simulink subsystem "Sensors"  (R2024b)
settings: Solver=VariableStepAuto  StartTime=0.0  StopTime=10.0  RelTol=1e-3
values from neighbouring files (symbols this model uses):
  CurrentFaultSwitch = 0    [Data__MOTOR.m]    (also in Generator_Data.m = 1; Generator_Datatest.m)
  rate_noise_i = 0.02*In    (= 0.22)    [Data__MOTOR.m]    (also in Generator_Data.m = 0.02; Generator_Datatest.m)
  rate_noise_w = 0.02*Wn    (= 2.96)    [Data__MOTOR.m]    (also in Generator_Data.m = 0.002; Generator_Datatest.m)
undefined symbols (not defined in the file or in its folder): sigbuilder_block
settings Model: Creator=Nasser  LastModifiedBy=Nasser

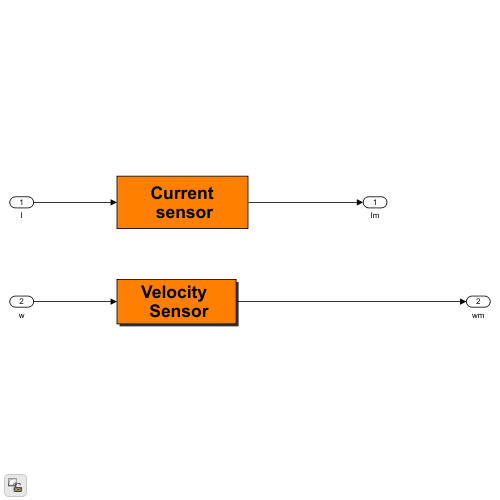
[thumbnail: Simulink's stored preview of the top-level diagram]
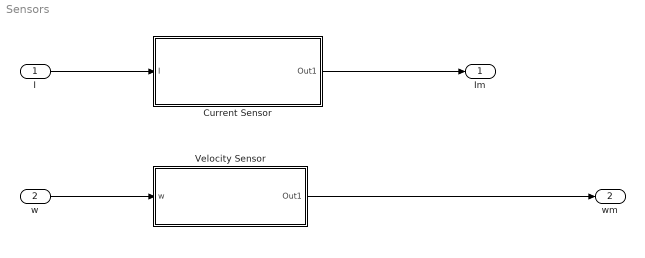
== system Sensors ==
  I : Inport
  w : Inport  Port=2
  Current Sensor : Subsystem
      mask Display: disp('Current\n sensor')
  Velocity Sensor : Subsystem
      mask Display: disp('Velocity \n Sensor')
  Im : Outport
  wm : Outport  Port=2
  wires:
  I/1 -> Current Sensor/1(I)
  w/1 -> Velocity Sensor/1(w)
  Current Sensor/1(Out1) -> Im/1
  Velocity Sensor/1(Out1) -> wm/1

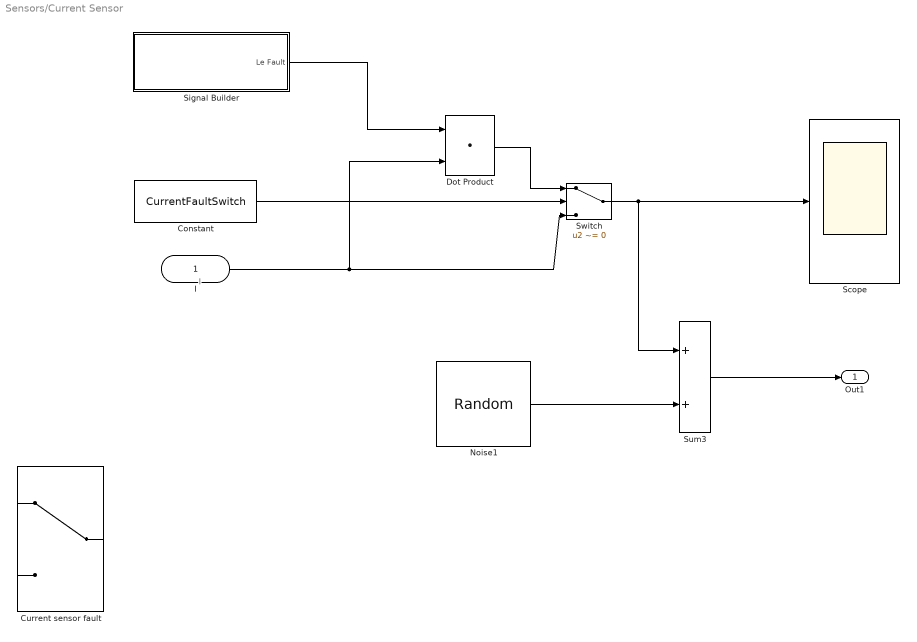
== system Sensors/Current Sensor ==
  note: I
  I : Inport
  Constant : Constant  Value=CurrentFaultSwitch
  Current sensor fault : ManualSwitch
  Dot Product : DotProduct  OutDataTypeStr=Inherit: Inherit via internal rule
  Noise1 : UniformRandomNumber  Minimum=-rate_noise_i  Maximum=+rate_noise_i  SampleTime=0.1
  Scope : Scope
  Signal Builder : Subsystem  Tag=STV Subsys  LoadFcn=sigbuilder_block('load');  StartFcn=sigbuilder_block('start');  StopFcn=sigbuilder_block('stop');  ClipboardFcn=sigbuilder_block('clipboard');  mask(Sigbuilder block){tuvar=[0:10]}
      mask help: Simulink:masks:SigbuilderBlock_MD
      mask init:
      | if ~strcmp(get_param(bdroot(gcbh),'SimulationStatus'),'stopped') tuvar = sigbuilder_block('maskInit'); end
      settings: CopyFcn=sigbuilder_block('copy');  DeleteFcn=sigbuilder_block('delete');  ModelCloseFcn=sigbuilder_block('modelClose');  PreSaveFcn=sigbuilder_block('preSave');  PauseFcn=sigbuilder_block('pause');  ContinueFcn=sigbuilder_block('continue');  NameChangeFcn=sigbuilder_block('namechange');  OpenFcn=sigbuilder_block('open',[1280 104 1024 485.5 ]);  CloseFcn=sigbuilder_block('close');
      mask Display: plot(0, 0, 100, 100,[2, 2, 32, 32, 2], [68, 8, 8, 68, 68],[32, 2], [38, 38], [32, 19, 2],[53, 60, 44], [32, 17, 17, 2],[16, 16, 31, 31]);txt = getActiveGroup(gcbh);text(2, 100, txt,'verticalAlignment', 'top');
  Sum3 : Sum  InputSameDT=on  SaturateOnIntegerOverflow=on  OutDataTypeStr=Inherit: Same as first input
  Switch : Switch  Criteria=u2 ~= 0  Threshold=1  SaturateOnIntegerOverflow=off  InputSameDT=off
  Out1 : Outport  VectorParamsAs1DForOutWhenUnconnected=off
  wires:
  Switch/1 -> Sum3/1, Scope/1
  Constant/1 -> Switch/2
  Dot Product/1 -> Switch/1
  Signal Builder/1(Le Fault) -> Dot Product/1
  I/1 -> Switch/3, Dot Product/2
  Noise1/1 -> Sum3/2
  Sum3/1 -> Out1/1

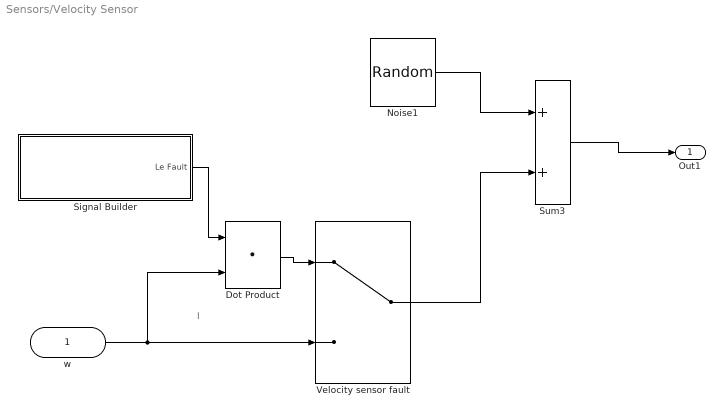
== system Sensors/Velocity Sensor ==
  note: I
  w : Inport
  Dot Product : DotProduct  OutDataTypeStr=Inherit: Inherit via internal rule
  Noise1 : UniformRandomNumber  Minimum=-rate_noise_w  Maximum=+rate_noise_w  SampleTime=0.1
  Signal Builder : Subsystem  Tag=STV Subsys  LoadFcn=sigbuilder_block('load');  StartFcn=sigbuilder_block('start');  StopFcn=sigbuilder_block('stop');  ClipboardFcn=sigbuilder_block('clipboard');  mask(Sigbuilder block){tuvar=[0:10]}
      mask help: Simulink:masks:SigbuilderBlock_MD
      mask init:
      | if ~strcmp(get_param(bdroot(gcbh),'SimulationStatus'),'stopped') tuvar = sigbuilder_block('maskInit'); end
      settings: CopyFcn=sigbuilder_block('copy');  DeleteFcn=sigbuilder_block('delete');  ModelCloseFcn=sigbuilder_block('modelClose');  PreSaveFcn=sigbuilder_block('preSave');  PauseFcn=sigbuilder_block('pause');  ContinueFcn=sigbuilder_block('continue');  NameChangeFcn=sigbuilder_block('namechange');  OpenFcn=sigbuilder_block('open',[122.4 104 1024.2 446.8 ]);  CloseFcn=sigbuilder_block('close');
      mask Display: plot(0, 0, 100, 100,[2, 2, 32, 32, 2], [68, 8, 8, 68, 68],[32, 2], [38, 38], [32, 19, 2],[53, 60, 44], [32, 17, 17, 2],[16, 16, 31, 31]);txt = getActiveGroup(gcbh);text(2, 100, txt,'verticalAlignment', 'top');
  Sum3 : Sum  InputSameDT=on  SaturateOnIntegerOverflow=on  OutDataTypeStr=Inherit: Same as first input
  Velocity sensor fault : ManualSwitch
  Out1 : Outport  VectorParamsAs1DForOutWhenUnconnected=off
  wires:
  Noise1/1 -> Sum3/1
  Velocity sensor fault/1 -> Sum3/2
  Dot Product/1 -> Velocity sensor fault/1
  Signal Builder/1(Le Fault) -> Dot Product/1
  w/1 -> Velocity sensor fault/2, Dot Product/2
  Sum3/1 -> Out1/1

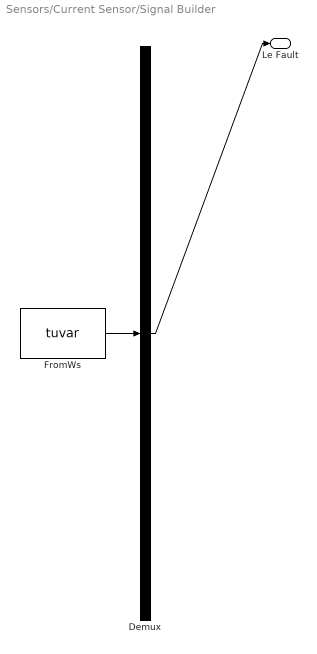
== system Sensors/Current Sensor/Signal Builder ==
  Demux : Demux  Tag=STV Demux  Outputs=1
      settings: DisplayOption=none
  FromWs : FromWorkspace  Tag=STV FromWs  VariableName=tuvar
      SigBuilderData=|
      | common.afterFinalStr = 'Extrapolate'
      | common.sampleTime = 0
      | dataSet.timeRange = [0 60]
      | dataSet.name = 'Group 1'
      | sbobj.Groups.Name = 'Group 1'
      | sbobj.Groups.Signals.Name = 'Le Fault'
      | sbobj.Groups.Signals.XData = [0 15.3 15.3 30.8 30.8 60]
      | sbobj.Groups.Signals.YData = [0.995 0.995 0.505 0.22 1 1]
      | sbobj.Groups.TimeRange = [0 60]
  Le Fault : Outport  Tag=STV Outport  VectorParamsAs1DForOutWhenUnconnected=off
  wires:
  Demux/1 -> Le Fault/1
  FromWs/1 -> Demux/1

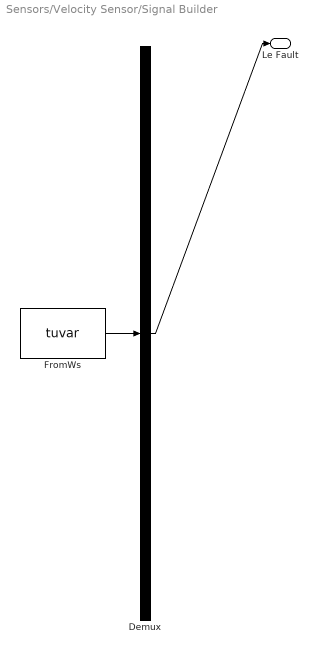
== system Sensors/Velocity Sensor/Signal Builder ==
  Demux : Demux  Tag=STV Demux  Outputs=1
      settings: DisplayOption=none
  FromWs : FromWorkspace  Tag=STV FromWs  VariableName=tuvar
      SigBuilderData=|
      | common.afterFinalStr = 'Extrapolate'
      | common.sampleTime = 0
      | dataSet.timeRange = [0 60]
      | dataSet.name = 'Group 1'
      | sbobj.Groups.Name = 'Group 1'
      | sbobj.Groups.Signals.Name = 'Le Fault'
      | sbobj.Groups.Signals.XData = [0 15.3 15.3 30.8 30.8 60]
      | sbobj.Groups.Signals.YData = [0.995 0.995 0.505 0.22 1 1]
      | sbobj.Groups.TimeRange = [0 60]
  Le Fault : Outport  Tag=STV Outport  VectorParamsAs1DForOutWhenUnconnected=off
  wires:
  Demux/1 -> Le Fault/1
  FromWs/1 -> Demux/1
